simulink model "P4p3"  (Simulink 8.3)
settings: Solver=ode1  StartTime=0.0  StopTime=inf  FixedStep=0.002  RelTol=1e-3
PostLoadFcn:
  | qc_set_target_type(getConfigSet(bdroot, 'QUARC Default Target Configuration'));
values from neighbouring files (symbols this model uses):
  A_se = [0 1 0 0 0 0 ... (first row only)    [P4p2_init.m]
  B_se = [0 0 ... (first row only)    [P4p2_init.m]
  C_se_no_pitch = [0 0 1 0 0 0 ... (first row only)    [P4p3_init.m]
  K_bar = lqr(A_bar, B_bar, Q_bar, R)    [P4p3_init.m]
  L = place(A_se', (C_se)', eigs_estimator)'    [P4p2_init.m]    (also in P4p2_integral_init.m = place(A_se', C_se', eigs_estimator_i)'; P4p3_init.m = place(A_se', C_se_no_pitch', eigs_estimator_i)')
  P = inv(C*inv(B*K - A)*B)    [P4p3_init.m]
  V_star = 6.5    [P4p2_init.m]
undefined symbols (not defined in the file or in its folder): E_OFF, HIL, Joystick_gain_x, Joystick_gain_y, P_OFF, qc_get_step_size, sigbuilder_block
libraries: simulink_extras x7, quarc_library x4
settings Model: Creator=Rchan  LastModifiedBy=bernharg  SimulationMode=external  ExtModeTrigDuration=5000
settings SolverCC: PositivePriorityOrder=on
settings OptimizationCC: ExpressionDepthLimit=2147483647  InitFltsAndDblsToZero=on
settings DebuggingCC: SaveWithParameterizedLinksMsg=none  MultiTaskDSMMsg=warning  MultiTaskCondExecSysMsg=none  FcnCallInpInsideContextMsg=EnableAllAsWarning  FrameProcessingCompatibilityMsg=error
settings RTWCC: SystemTargetFile=quarc_win64.tlc  TemplateMakefile=quarc_default_tmf  Description=QUARC Win64 Target  ProcessScript=quarc_win64_make_rtw_hook
settings STFCustomTargetCC: TargetPreCompLibLocation=C:\PROGRA~3\QUARC\lib\2014a\win64\release  ConcurrentExecutionCompliant=on  GeneratePreprocessorConditionals=Disable all  CPPClassGenCompliant=on  SystemTargetFile=quarc_win64.tlc
settings GRTTargetCC: TargetPreCompLibLocation=C:\PROGRA~3\QUARC\lib\2014a\win64\release  ParMdlRefBuildCompliant=off  CompOptLevelCompliant=off  MatFileLogging=off  ExtMode=on  ExtModeMexFile=quarc_comm

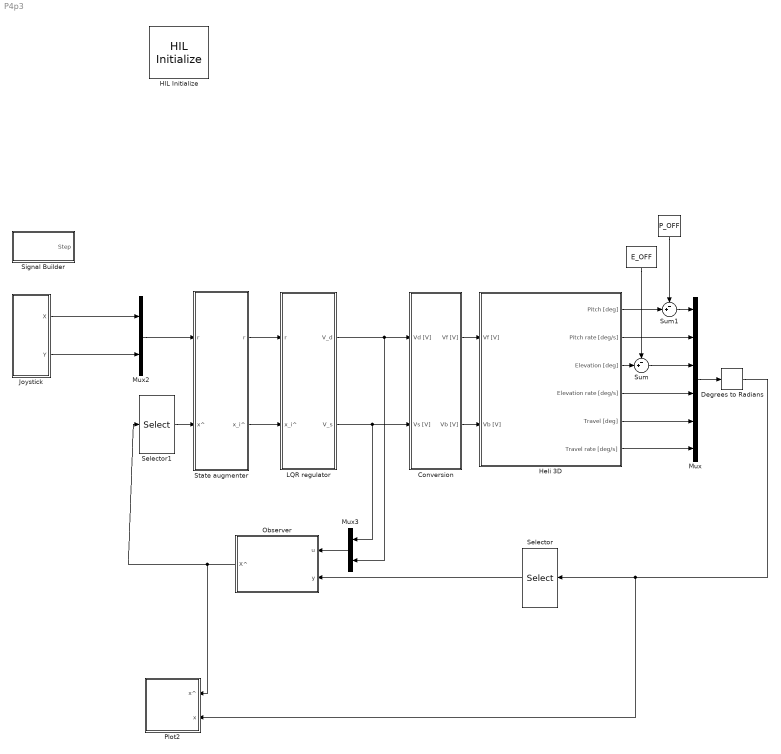
== system P4p3 ==
  "   " : Constant  Value=P_OFF
  "     " : Constant  Value=E_OFF
  Conversion : Subsystem
  Degrees to Radians : simulink_extras/Transformations/Degrees to Radians
  HIL Initialize : quarc_library/Data Acquisition/Generic/Configuration/HIL Initialize  Priority=-99  object_name=HIL-1  board_type=q8_usb  board_number=0  board_options=update_rate=normal;decimation=1  exclusive=off  active=off  hardware_clocks=[0:2]  clock_modes=[]  initial_clock_frequencies=[]  set_clock_params_at_start=off  set_clock_params_at_switch_in=off  set_clock_frequencies_at_start=off  set_clock_frequencies_at_switch_in=off  analog_input_channels=[0:7]  analog_input_maximums=10  analog_input_minimums=-10  set_analog_input_params_at_start=on  set_analog_input_params_at_switch_in=off  analog_output_channels=[0:7]  analog_output_maximums=10  analog_output_minimums=-10  initial_analog_outputs=[0]  final_analog_outputs=[0]  watchdog_analog_outputs=0  set_analog_output_params_at_start=on  set_analog_output_params_at_switch_in=off  set_analog_outputs_at_start=on  set_analog_outputs_at_switch_in=off  set_analog_outputs_at_terminate=on  set_analog_outputs_at_switch_out=off  set_analog_outputs_on_watchdog=off  digital_input_channels=[]  digital_output_channels=[]  digital_output_configuration=[]  initial_digital_outputs=[1]  final_digital_outputs=[1]  watchdog_digital_outputs=[1]  set_digital_output_params_at_start=off  set_digital_output_params_at_switch_in=off  set_digital_outputs_at_start=on  set_digital_outputs_at_switch_in=off  set_digital_outputs_at_terminate=on  set_digital_outputs_at_switch_out=off  set_digital_outputs_on_watchdog=off  encoder_channels=[0:7]  quadrature=[4]  encoder_filter_frequency=[]  initial_encoder_counts=[0]  set_encoder_params_at_start=on  set_encoder_params_at_switch_in=off  set_encoder_counts_at_start=on  set_encoder_counts_at_switch_in=off  pwm_channels=[0:7]  pwm_modes=0  pwm_frequency=99.532799999999995e6/4095  pwm_configuration=[0]  pwm_alignment=[0]  pwm_polarity=[1]  pwm_leading_deadband=[0]  pwm_trailing_deadband=[0]  initial_pwm_outputs=[0]  final_pwm_outputs=[0]  watchdog_pwm_outputs=[0]  set_pwm_params_at_start=on  set_pwm_params_at_switch_in=off  set_pwm_outputs_at_start=on  set_pwm_outputs_at_switch_in=off  set_pwm_outputs_at_terminate=on  set_pwm_outputs_at_switch_out=off  set_pwm_outputs_on_watchdog=off  other_output_channels=[]  initial_other_outputs=[]  final_other_outputs=[]  watchdog_other_outputs=[]  set_other_outputs_at_start=off  set_other_outputs_at_switch_in=off  set_other_outputs_at_terminate=off  set_other_outputs_at_switch_out=off  set_other_outputs_on_watchdog=off
  Heli 3D : Subsystem
  Joystick : Subsystem
  LQR regulator : Subsystem
  Mux : Mux  Inputs=6
  Mux2 : Mux  Inputs=2
  Mux3 : Mux  Inputs=2
  Observer : Subsystem
  Plot2 : Subsystem
  Selector : Selector  InputPortWidth=6  Indices=[3 5]
  Selector1 : Selector  InputPortWidth=6  Indices=[1 2 4]
  Signal Builder : Subsystem  Tag=STV Subsys  LoadFcn=sigbuilder_block('load');  StartFcn=sigbuilder_block('start');  StopFcn=sigbuilder_block('stop');  ClipboardFcn=sigbuilder_block('clipboard');  mask(Sigbuilder block){}
      mask help: Simulink:masks:SigbuilderBlock_MD
      mask init:
      | if ~strcmp(get_param(bdroot(gcbh),'SimulationStatus'),'stopped') tuvar = sigbuilder_block('maskInit'); end
      settings: CopyFcn=sigbuilder_block('copy');  DeleteFcn=sigbuilder_block('delete');  ModelCloseFcn=sigbuilder_block('modelClose');  PreSaveFcn=sigbuilder_block('preSave');  PauseFcn=sigbuilder_block('pause');  ContinueFcn=sigbuilder_block('continue');  NameChangeFcn=sigbuilder_block('namechange');  OpenFcn=sigbuilder_block('open',[437.25 199.5 550.5 399.75 ]);  CloseFcn=sigbuilder_block('close');
      mask Display: plot(0, 0, 100, 100,[2, 2, 32, 32, 2], [68, 8, 8, 68, 68],[32, 2], [38, 38], [32, 19, 2],[53, 60, 44], [32, 17, 17, 2],[16, 16, 31, 31]);txt = getActiveGroup(gcbh);text(2, 100, txt,'verticalAlignment', 'top');
  State augmenter : Subsystem
  Sum : Sum  Inputs=-+|
  Sum1 : Sum  Inputs=-+|
  wires:
  Conversion/1(Vf [V]) -> Heli 3D/1(Vf [V])
  Conversion/2(Vb [V]) -> Heli 3D/2(Vb [V])
  Mux2/1 -> State augmenter/1(r)
  LQR regulator/1(V_d) -> Mux3/2, Conversion/1(Vd [V])
  LQR regulator/2(V_s) -> Mux3/1, Conversion/2(Vs [V])
  Mux/1 -> Degrees to Radians/1
  Heli 3D/2(Pitch rate [deg/s]) -> Mux/2
  Heli 3D/5(Travel [deg]) -> Mux/5
  Heli 3D/6(Travel rate [deg/s]) -> Mux/6
  Heli 3D/4(Elevation rate [deg/s]) -> Mux/4
  "     "/1 -> Sum/1
  Heli 3D/3(Elevation [deg]) -> Sum/2
  Sum/1 -> Mux/3
  Heli 3D/1(Pitch [deg]) -> Sum1/2
  "   "/1 -> Sum1/1
  Sum1/1 -> Mux/1
  Mux3/1 -> Observer/1(u)
  Degrees to Radians/1 -> Plot2/2(x), Selector/1
  Selector/1 -> Observer/2(y)
  Observer/1(X^) -> Plot2/1(x^), Selector1/1
  State augmenter/2("x_i^ ") -> LQR regulator/2(x_i^)
  State augmenter/1("r  ") -> LQR regulator/1(r)
  Selector1/1 -> State augmenter/2(x^)
  Joystick/1(X) -> Mux2/1
  Joystick/2(Y) -> Mux2/2

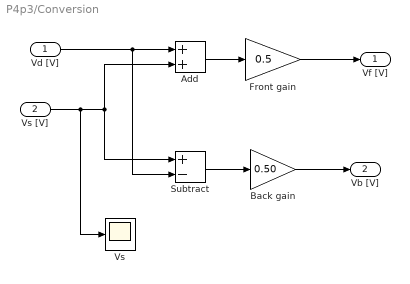
== system P4p3/Conversion ==
  Vd [V] : Inport
  Vs [V] : Inport  Port=2
  Add : Sum
  Back gain : Gain  Gain=0.50
  Front gain : Gain  Gain=0.5
  Subtract : Sum  Inputs=+-
  Vs : Scope
      settings: YMin=-0  YMax=6.5
  Vf [V] : Outport
  Vb [V] : Outport  Port=2
  wires:
  Vd [V]/1 -> Subtract/2, Add/1
  Vs [V]/1 -> Vs/1, Subtract/1, Add/2
  Subtract/1 -> Back gain/1
  Back gain/1 -> Vb [V]/1
  Add/1 -> Front gain/1
  Front gain/1 -> Vf [V]/1

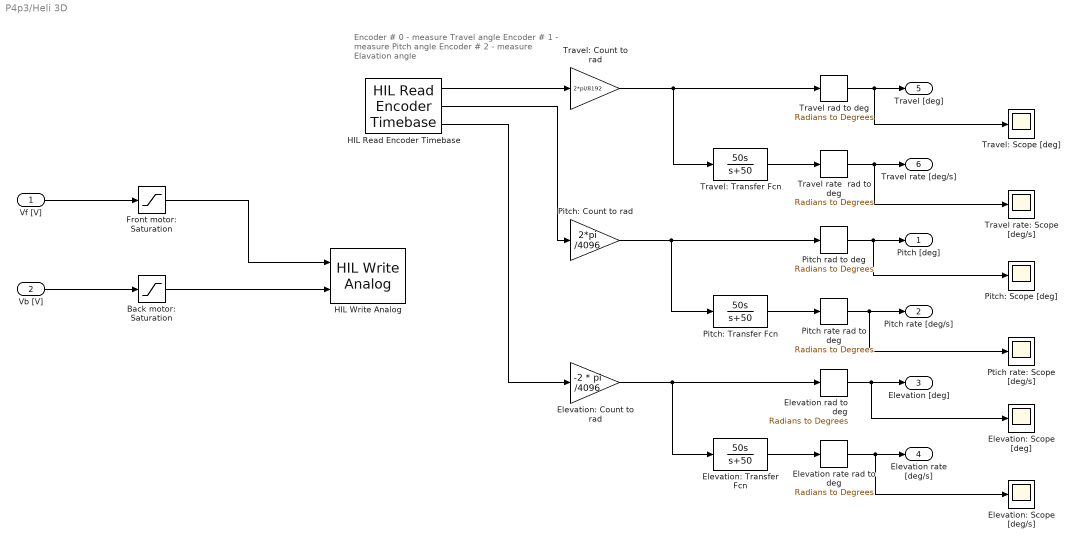
== system P4p3/Heli 3D ==
  note: Encoder # 0 - measure Travel angle
      | Encoder # 1 - measure Pitch angle
      | Encoder # 2 - measure Elavation angle
  Vf [V] : Inport
  Vb [V] : Inport  Port=2
  Back motor: Saturation : Saturate  UpperLimit=5  LowerLimit=-5
  Elevation rad to deg : simulink_extras/Transformations/Radians to Degrees
  Elevation rate rad to deg : simulink_extras/Transformations/Radians to Degrees
  Elevation: Count to rad : Gain  Gain=-2 * pi /4096
  Elevation: Scope [deg/s] : Scope
      settings: YMin=-15  YMax=15  SaveName=ScopeData13
  Elevation: Scope [deg] : Scope
      settings: YMin=-30  YMax=12.5  SaveName=ScopeData12
  Elevation: Transfer Fcn : TransferFcn  Numerator=[50 0]  Denominator=[1 50]
  Front motor: Saturation : Saturate  UpperLimit=5  LowerLimit=-5
  HIL Read Encoder Timebase : quarc_library/Data Acquisition/Generic/Timebases/HIL Read Encoder Timebase  object_name=HIL-1  clock=0  channels=[0:2]  samples_in_buffer=max(ceil(1/qc_get_step_size), 1)  active=on  vector_output=off  data_type_mode=Inherit via back propagation  data_type=double
  HIL Write Analog : quarc_library/Data Acquisition/Generic/Immediate I//O/HIL Write Analog  object_name=HIL-1  channels=[0:1]  sample_time=-1  active=off  vector_input=off
  Pitch rad to deg : simulink_extras/Transformations/Radians to Degrees
  Pitch rate rad to deg : simulink_extras/Transformations/Radians to Degrees
  Pitch: Count to rad : Gain  Gain=2*pi /4096
  Pitch: Scope [deg] : Scope
      settings: YMin=-1.3  YMax=0  SaveName=ScopeData10
  Pitch: Transfer Fcn : TransferFcn  Numerator=[50 0]  Denominator=[1 50]
  Ptich rate: Scope [deg/s] : Scope
      settings: YMin=-15  YMax=15  SaveName=ScopeData11
  Travel rad to deg : simulink_extras/Transformations/Radians to Degrees
  Travel rate  rad to deg : simulink_extras/Transformations/Radians to Degrees
  Travel rate: Scope [deg/s] : Scope
      settings: YMin=-15  YMax=15  SaveName=ScopeData9
  Travel: Count to rad : Gain  Gain=2*pi/8192
  Travel: Scope [deg] : Scope
      settings: YMin=-15  YMax=15  SaveName=ScopeData8
  Travel: Transfer Fcn : TransferFcn  Numerator=[50 0]  Denominator=[1 50]
  Pitch [deg] : Outport
  Pitch rate [deg/s] : Outport  Port=2
  Elevation [deg] : Outport  Port=3
  Elevation rate [deg/s] : Outport  Port=4
  Travel [deg] : Outport  Port=5
  Travel rate [deg/s] : Outport  Port=6
  wires:
  HIL Read Encoder Timebase/1 -> Travel: Count to rad/1
  HIL Read Encoder Timebase/3 -> Elevation: Count to rad/1
  Travel: Count to rad/1 -> Travel: Transfer Fcn/1, Travel rad to deg/1
  Travel: Transfer Fcn/1 -> Travel rate  rad to deg/1
  Pitch: Count to rad/1 -> Pitch: Transfer Fcn/1, Pitch rad to deg/1
  Pitch: Transfer Fcn/1 -> Pitch rate rad to deg/1
  Elevation: Count to rad/1 -> Elevation: Transfer Fcn/1, Elevation rad to deg/1
  Elevation: Transfer Fcn/1 -> Elevation rate rad to deg/1
  Travel rad to deg/1 -> Travel: Scope [deg]/1, Travel [deg]/1
  Travel rate  rad to deg/1 -> Travel rate: Scope [deg/s]/1, Travel rate [deg/s]/1
  Pitch rad to deg/1 -> Pitch: Scope [deg]/1, Pitch [deg]/1
  Pitch rate rad to deg/1 -> Ptich rate: Scope [deg/s]/1, Pitch rate [deg/s]/1
  Elevation rate rad to deg/1 -> Elevation: Scope [deg/s]/1, Elevation rate [deg/s]/1
  Vf [V]/1 -> Front motor: Saturation/1
  Vb [V]/1 -> Back motor: Saturation/1
  Front motor: Saturation/1 -> HIL Write Analog/1
  Back motor: Saturation/1 -> HIL Write Analog/2
  Elevation rad to deg/1 -> Elevation [deg]/1, Elevation: Scope [deg]/1
  HIL Read Encoder Timebase/2 -> Pitch: Count to rad/1

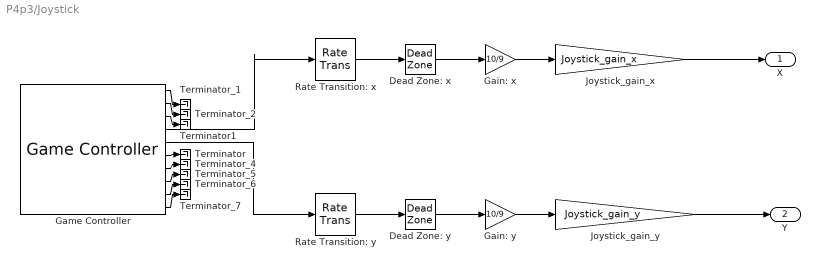
== system P4p3/Joystick ==
  Dead Zone: x : DeadZone  LowerValue=-0.1  UpperValue=0.1  SaturateOnIntegerOverflow=on
  Dead Zone: y : DeadZone  LowerValue=-0.1  UpperValue=0.1  SaturateOnIntegerOverflow=on
  Gain: x : Gain  Gain=10/9
  Gain: y : Gain  Gain=10/9
  Game Controller : quarc_library/Devices/Peripherals/Target/Game Controller  controller=1  buffer_size=12  deadzone=[]  saturation=[]  sample_time=max(qc_get_step_size, 0.01)  auto_center=off  enabled=on
  Joystick_gain_x : Gain  Gain=Joystick_gain_x
  Joystick_gain_y : Gain  Gain=Joystick_gain_y
  Rate Transition: x : RateTransition
  Rate Transition: y : RateTransition
  Terminator : Terminator
  Terminator1 : Terminator
  Terminator_{1..2,4..7} (6 alike) : Terminator
  X : Outport
  Y : Outport  Port=2
  wires:
  Rate Transition: y/1 -> Dead Zone: y/1
  Rate Transition: x/1 -> Dead Zone: x/1
  Game Controller/5 -> Rate Transition: y/1
  Game Controller/4 -> Rate Transition: x/1
  Game Controller/1 -> Terminator_1/1
  Game Controller/2 -> Terminator_2/1
  Game Controller/7 -> Terminator_4/1
  Game Controller/8 -> Terminator_5/1
  Game Controller/9 -> Terminator_6/1
  Game Controller/10 -> Terminator_7/1
  Game Controller/3 -> Terminator1/1
  Game Controller/6 -> Terminator/1
  Dead Zone: x/1 -> Gain: x/1
  Dead Zone: y/1 -> Gain: y/1
  Gain: x/1 -> Joystick_gain_x/1
  Gain: y/1 -> Joystick_gain_y/1
  Joystick_gain_x/1 -> X/1
  Joystick_gain_y/1 -> Y/1

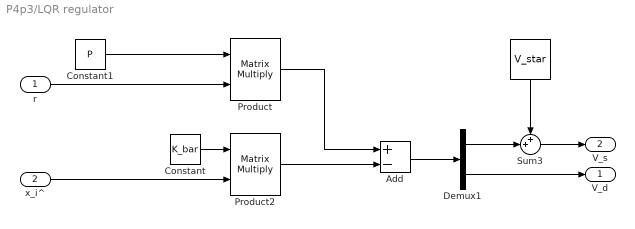
== system P4p3/LQR regulator ==
  r : Inport
  x_i^ : Inport  Port=2
  " " : Constant  Value=V_star
  Add : Sum  Inputs=+-
  Constant : Constant  Value=K_bar
  Constant1 : Constant  Value=P
  Demux1 : Demux  Outputs=2
  Product : Product  Multiplication=Matrix(*)
  Product2 : Product  Multiplication=Matrix(*)
  Sum3 : Sum  Inputs=++|
  V_d : Outport
  V_s : Outport  Port=2
  wires:
  Demux1/2 -> V_d/1
  Constant1/1 -> Product/1
  Product/1 -> Add/1
  Add/1 -> Demux1/1
  Sum3/1 -> V_s/1
  " "/1 -> Sum3/1
  Demux1/1 -> Sum3/2
  Constant/1 -> Product2/1
  Product2/1 -> Add/2
  r/1 -> Product/2
  x_i^/1 -> Product2/2

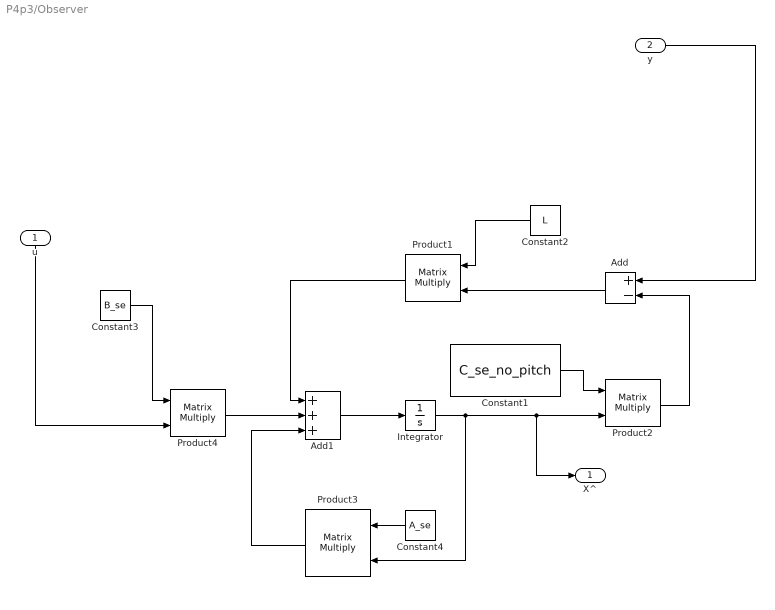
== system P4p3/Observer ==
  u : Inport
  y : Inport  Port=2
  Add : Sum  Inputs=+-
  Add1 : Sum  Inputs=+++
  Constant1 : Constant  Value=C_se_no_pitch
  Constant2 : Constant  Value=L
  Constant3 : Constant  Value=B_se
  Constant4 : Constant  Value=A_se
  Integrator : Integrator
  Product{1..4} (4 alike) : Product  Multiplication=Matrix(*)
  X^ : Outport
  wires:
  Product2/1 -> Add/2
  Add1/1 -> Integrator/1
  Add/1 -> Product1/2
  Product4/1 -> Add1/2
  u/1 -> Product4/2
  Integrator/1 -> Product3/2, Product2/2, X^/1
  y/1 -> Add/1
  Product1/1 -> Add1/1
  Product3/1 -> Add1/3
  Constant3/1 -> Product4/1
  Constant4/1 -> Product3/1
  Constant1/1 -> Product2/1
  Constant2/1 -> Product1/1

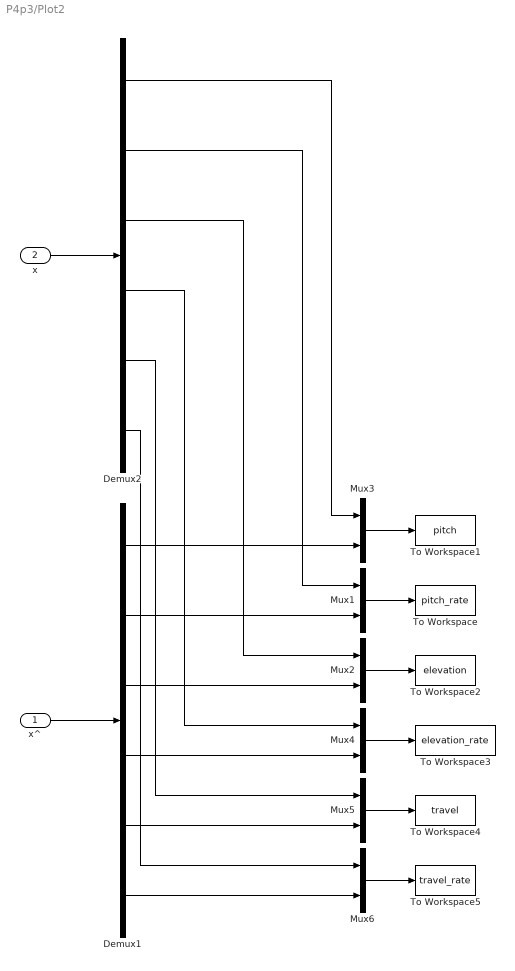
== system P4p3/Plot2 ==
  x^ : Inport
  x : Inport  Port=2
  Demux1 : Demux  Outputs=6
  Demux2 : Demux  Outputs=6
  Mux{1..6} (6 alike) : Mux  Inputs=2
  To Workspace : ToWorkspace  VariableName=pitch_rate  SampleTime=-1
  To Workspace1 : ToWorkspace  VariableName=pitch  SampleTime=-1
  To Workspace2 : ToWorkspace  VariableName=elevation  SampleTime=-1
  To Workspace3 : ToWorkspace  VariableName=elevation_rate  SampleTime=-1
  To Workspace4 : ToWorkspace  VariableName=travel  SampleTime=-1
  To Workspace5 : ToWorkspace  VariableName=travel_rate  SampleTime=-1
  wires:
  Mux1/1 -> To Workspace/1
  Mux3/1 -> To Workspace1/1
  x/1 -> Demux2/1
  x^/1 -> Demux1/1
  Demux1/1 -> Mux3/2
  Mux2/1 -> To Workspace2/1
  Mux4/1 -> To Workspace3/1
  Mux5/1 -> To Workspace4/1
  Mux6/1 -> To Workspace5/1
  Demux1/2 -> Mux1/2
  Demux1/3 -> Mux2/2
  Demux1/4 -> Mux4/2
  Demux1/5 -> Mux5/2
  Demux1/6 -> Mux6/2
  Demux2/1 -> Mux3/1
  Demux2/2 -> Mux1/1
  Demux2/3 -> Mux2/1
  Demux2/4 -> Mux4/1
  Demux2/5 -> Mux5/1
  Demux2/6 -> Mux6/1

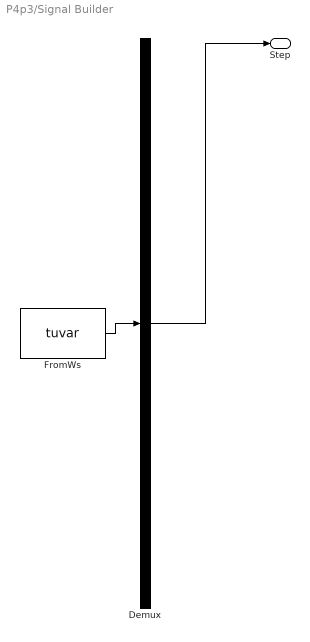
== system P4p3/Signal Builder ==
  Demux : Demux  Tag=STV Demux  Outputs=1
  FromWs : FromWorkspace  Tag=STV FromWs  VariableName=tuvar  SampleTime=0  SigBuilderData=DataTag3  VnvData=DataTag4
      SigBuilderData=|
      | common.afterFinalStr = 'Extrapolate'
      | common.sampleTime = 0
      | dataSet.timeRange = [0 10]
      | dataSet.name = 'Group 1'
      | sbobj.Groups.Name = 'Group 1'
      | sbobj.Groups.Signals.Name = 'Step'
      | sbobj.Groups.Signals.XData = [0 4 4 8.02 8.02 10]
      | sbobj.Groups.Signals.YData = [0 -0.002 0.465 0.465 0 0]
  Step : Outport  Tag=STV Outport
  wires:
  Demux/1 -> Step/1
  FromWs/1 -> Demux/1

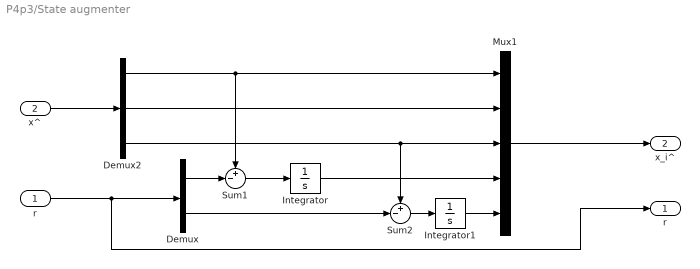
== system P4p3/State augmenter ==
  r : Inport
  x^ : Inport  Port=2
  Demux : Demux  Outputs=2
  Demux2 : Demux  Outputs=3
  Integrator : Integrator
  Integrator1 : Integrator
  Mux1 : Mux  Inputs=5
  Sum1 : Sum  Inputs=+-|
  Sum2 : Sum  Inputs=+-|
  "r  " : Outport
  "x_i^ " : Outport  Port=2
  wires:
  r/1 -> "r  "/1, Demux/1
  x^/1 -> Demux2/1
  Sum1/1 -> Integrator/1
  Integrator/1 -> Mux1/4
  Sum2/1 -> Integrator1/1
  Integrator1/1 -> Mux1/5
  Demux/1 -> Sum1/2
  Demux/2 -> Sum2/2
  Demux2/1 -> Mux1/1, Sum1/1
  Demux2/3 -> Sum2/1, Mux1/3
  Demux2/2 -> Mux1/2
  Mux1/1 -> "x_i^ "/1
